simulink model "paperJournalofProcessControl_Model"  (Simulink 7.7)
settings: Solver=ode45  StartTime=0.0  StopTime=1.5  RelTol=1e-3
libraries: cstblocks x11
settings Model: Creator=kostis  LastModifiedBy=kostis

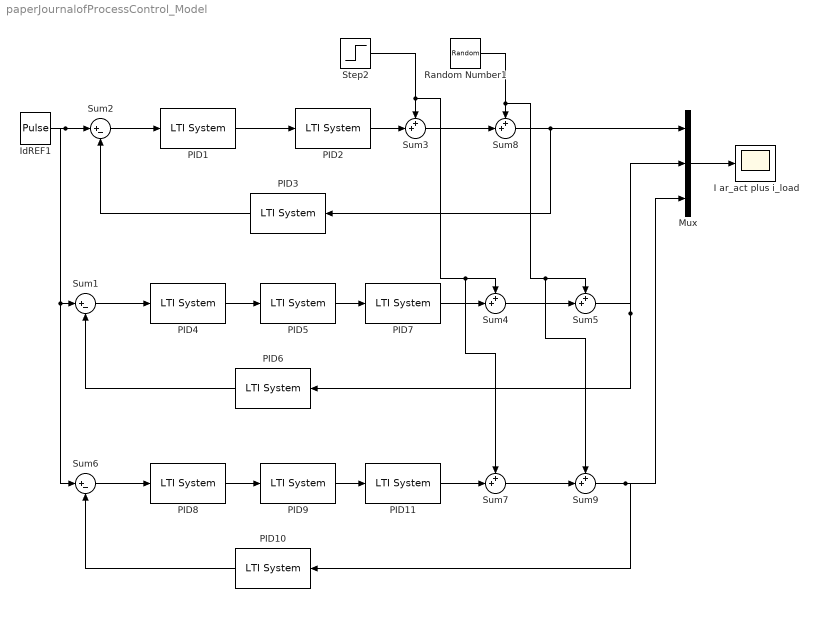
== system paperJournalofProcessControl_Model ==
  I ar_act plus i_load : Scope
      settings: TickLabels=on  TimeRange=0.6000000000000001  YMin=0.95  YMax=1.75  SaveName=OutputSignal  SampleInput=on  SampleTime=0.001
  IdREF1 : DiscretePulseGenerator  PulseType=Time based  Period=10  PulseWidth=50  PhaseDelay=0.35
  Mux : Mux  Inputs=3
  PID1 : cstblocks/LTI System  SystemSampleTime=-1  sys=Gc  IC=[]
  PID10 : cstblocks/LTI System  SystemSampleTime=-1  sys=kh  IC=[]
  PID11 : cstblocks/LTI System  SystemSampleTime=-1  sys=Gp_NET_2  IC=[]
  PID2 : cstblocks/LTI System  SystemSampleTime=-1  sys=Gp  IC=[]
  PID3 : cstblocks/LTI System  SystemSampleTime=-1  sys=kh  IC=[]
  PID4 : cstblocks/LTI System  SystemSampleTime=-1  sys=Gc  IC=[]
  PID5 : cstblocks/LTI System  SystemSampleTime=-1  sys=Gp  IC=[]
  PID6 : cstblocks/LTI System  SystemSampleTime=-1  sys=kh  IC=[]
  PID7 : cstblocks/LTI System  SystemSampleTime=-1  sys=Gp_NET  IC=[]
  PID8 : cstblocks/LTI System  SystemSampleTime=-1  sys=Gc  IC=[]
  PID9 : cstblocks/LTI System  SystemSampleTime=-1  sys=Gp  IC=[]
  Random Number1 : RandomNumber  Variance=0.00005  Seed=0.0025  SampleTime=0.00001
  Step2 : Step  Time=0.75  After=0.7  SampleTime=0
  Sum1 : Sum  Inputs=|+-
  Sum2 : Sum  Inputs=|+-
  Sum{3..5,7..9} (6 alike) : Sum  Inputs=++|
  Sum6 : Sum  Inputs=|+-
  wires:
  PID2/1 -> Sum3/2
  Step2/1 -> Sum3/1, Sum4/1, Sum7/1
  Sum3/1 -> Sum8/2
  Random Number1/1 -> Sum8/1, Sum5/1, Sum9/1
  Sum8/1 -> PID3/1, Mux/1
  PID1/1 -> PID2/1
  PID3/1 -> Sum2/2
  Sum2/1 -> PID1/1
  IdREF1/1 -> Sum2/1, Sum1/1, Sum6/1
  Sum4/1 -> Sum5/2
  Sum5/1 -> PID6/1, Mux/2
  PID4/1 -> PID5/1
  PID6/1 -> Sum1/2
  Sum1/1 -> PID4/1
  Mux/1 -> I ar_act plus i_load/1
  PID7/1 -> Sum4/2
  PID5/1 -> PID7/1
  Sum7/1 -> Sum9/2
  Sum9/1 -> PID10/1, Mux/3
  PID8/1 -> PID9/1
  PID10/1 -> Sum6/2
  Sum6/1 -> PID8/1
  PID11/1 -> Sum7/2
  PID9/1 -> PID11/1
